simulink model "Testbed_v3"  (R2020a)
settings: Solver=ode23tb  StartTime=0.0  StopTime=20  MaxStep=0.066666666666666671  RelTol=1e-4  EnableMultiTasking=on
undefined symbols (not defined in the file): D11, Delta
libraries: powerlib x95, dspnetwork x75, dspstat3 x52, eePMU x16
(part 1 of 2)
settings Model: SimulationMode=accelerator  PacingRate=2000  Creator=vaibhav  LastModifiedBy=ray
settings SolverCC: MaxConsecutiveZCs=10000  ZeroCrossControl=EnableAll  ZeroCrossAlgorithm=Adaptive  SolverResetMethod=Robust
settings DataIOCC: LimitDataPoints=on  SaveFormat=Array  ReturnWorkspaceOutputs=off
settings OptimizationCC: ExpressionDepthLimit=2147483647  LifeSpan=inf
settings DebuggingCC: UnderspecifiedInitializationDetection=Classic  MergeDetectMultiDrivingBlocksExec=none  MaskedZcDiagnostic=none  IgnoredZcDiagnostic=none  SolverPrmCheckMsg=warning  FcnCallInpInsideContextMsg=warning  StateNameClashWarn=warning  SFUnexpectedBacktrackingDiag=warning  SFNoUnconditionalDefaultTransitionDiag=warning  SFExecutionAtInitializationDiag=none  ArithmeticOperatorsInVariantConditions=warning
settings HardwareCC: ProdBitPerPointer=32  ProdBitPerSizeT=32  ProdBitPerPtrDiffT=32  ProdLargestAtomicFloat=None  ProdIntDivRoundTo=Undefined  ProdEndianess=Unspecified  ProdWordSize=32  ProdHWDeviceType=32-bit Generic
settings ModelReferenceCC: PropagateSignalLabelsOutOfModel=off
settings SFSimCC: SimUseLocalCustomCode=off  CustomCodeUndefinedFunction=UseInterfaceOnly
settings RTWCC: RTWUseLocalCustomCode=off
settings CodeAppCC: StateflowObjectComments=on
settings GRTTargetCC: TargetLangStandard=C89/C90 (ANSI)  CombineOutputUpdateFcns=off  GRTInterface=on
settings ConfigComp: CovMetricSettings=dw  CovHtmlReporting=on  CovSaveCumulativeToWorkspaceVar=on  CovSaveSingleToWorkspaceVar=on  CovExternalEMLEnable=off

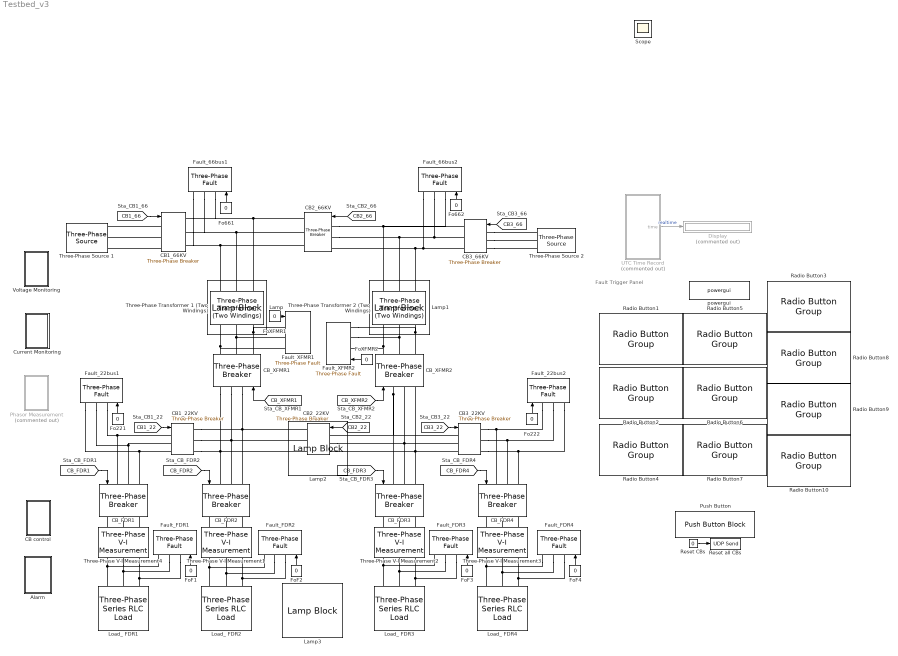
== system Testbed_v3 ==
  note: Fault Trigger
      | Panel
  Alarm : Subsystem
  CB control : Subsystem
  CB1_22KV : powerlib/Elements/Three-Phase Breaker  InitialState=closed  SwitchA=on  SwitchB=on  SwitchC=on  SwitchTimes="[1/10  2/10]"  External=on  BreakerResistance=0.0001  SnubberResistance=inf  SnubberCapacitance=inf  Measurements=Breaker voltages and currents
  CB1_66KV : powerlib/Elements/Three-Phase Breaker  InitialState=closed  SwitchA=on  SwitchB=on  SwitchC=on  SwitchTimes="[1/10  2/10]"  External=on  BreakerResistance=0.0001  SnubberResistance=inf  SnubberCapacitance=inf  Measurements=Breaker voltages and currents
  CB2_22KV : powerlib/Elements/Three-Phase Breaker  InitialState=closed  SwitchA=on  SwitchB=on  SwitchC=on  SwitchTimes="[1/10  2/10]"  External=on  BreakerResistance=0.0001  SnubberResistance=inf  SnubberCapacitance=inf  Measurements=Breaker voltages and currents
  CB2_66KV : powerlib/Elements/Three-Phase Breaker  InitialState=closed  SwitchA=on  SwitchB=on  SwitchC=on  SwitchTimes="[1/10  2/10]"  External=on  BreakerResistance=0.0001  SnubberResistance=inf  SnubberCapacitance=inf  Measurements=Breaker voltages and currents
  CB3_22KV : powerlib/Elements/Three-Phase Breaker  InitialState=closed  SwitchA=on  SwitchB=on  SwitchC=on  SwitchTimes="[1/10  2/10]"  External=on  BreakerResistance=0.0001  SnubberResistance=inf  SnubberCapacitance=inf  Measurements=Breaker voltages and currents
  CB3_66KV : powerlib/Elements/Three-Phase Breaker  InitialState=closed  SwitchA=on  SwitchB=on  SwitchC=on  SwitchTimes="[1/10  2/10]"  External=on  BreakerResistance=0.0001  SnubberResistance=inf  SnubberCapacitance=inf  Measurements=Breaker voltages and currents
  CB_FDR{1..4} (4 alike) : powerlib/Elements/Three-Phase Breaker  InitialState=closed  SwitchA=on  SwitchB=on  SwitchC=on  SwitchTimes="[1/10  2/10]"  External=on  BreakerResistance=0.0001  SnubberResistance=inf  SnubberCapacitance=inf  Measurements=Breaker voltages and currents
  CB_XFMR1 : powerlib/Elements/Three-Phase Breaker  InitialState=closed  SwitchA=on  SwitchB=on  SwitchC=on  SwitchTimes="[1/10  2/10]"  External=on  BreakerResistance=0.0001  SnubberResistance=inf  SnubberCapacitance=inf  Measurements=Breaker voltages and currents
  CB_XFMR2 : powerlib/Elements/Three-Phase Breaker  InitialState=closed  SwitchA=on  SwitchB=on  SwitchC=on  SwitchTimes="[1/10  2/10]"  External=on  BreakerResistance=0.0001  SnubberResistance=inf  SnubberCapacitance=inf  Measurements=Breaker voltages and currents
  Current Monitoring : Subsystem
  Display : Display  Commented=on
  Fault_22bus1 : powerlib/Elements/Three-Phase Fault  InitialStates=0  FaultA=on  FaultB=on  FaultC=on  GroundFault=off  SwitchTimes="[1/60  5/60]"  External=on  SwitchStatus=NaN  FaultResistance=0.0001  GroundResistance=0.01  SnubberResistance=inf  SnubberCapacitance=inf  Measurements=Fault voltages and currents
  Fault_22bus2 : powerlib/Elements/Three-Phase Fault  InitialStates=0  FaultA=on  FaultB=on  FaultC=on  GroundFault=off  SwitchTimes="[1/60  5/60]"  External=on  SwitchStatus=NaN  FaultResistance=0.0001  GroundResistance=0.01  SnubberResistance=inf  SnubberCapacitance=inf  Measurements=Fault voltages and currents
  Fault_66bus1 : powerlib/Elements/Three-Phase Fault  InitialStates=0  FaultA=on  FaultB=on  FaultC=on  GroundFault=off  SwitchTimes="[1/60  5/60]"  External=on  SwitchStatus=NaN  FaultResistance=0.0001  GroundResistance=0.01  SnubberResistance=inf  SnubberCapacitance=inf  Measurements=Fault voltages and currents
  Fault_66bus2 : powerlib/Elements/Three-Phase Fault  InitialStates=0  FaultA=on  FaultB=on  FaultC=on  GroundFault=off  SwitchTimes="[1/60  5/60]"  External=on  SwitchStatus=NaN  FaultResistance=0.0001  GroundResistance=0.01  SnubberResistance=inf  SnubberCapacitance=inf  Measurements=Fault voltages and currents
  Fault_FDR{1..4} (4 alike) : powerlib/Elements/Three-Phase Fault  InitialStates=0  FaultA=on  FaultB=on  FaultC=on  GroundFault=off  SwitchTimes="[1/60  5/60]"  External=on  SwitchStatus=NaN  FaultResistance=0.0001  GroundResistance=0.00001  SnubberResistance=inf  SnubberCapacitance=inf  Measurements=Fault voltages and currents
  Fault_XFMR1 : powerlib/Elements/Three-Phase Fault  InitialStates=0  FaultA=on  FaultB=on  FaultC=on  GroundFault=off  SwitchTimes="[1/60  5/60]"  External=on  SwitchStatus=NaN  FaultResistance=0.0001  GroundResistance=0.01  SnubberResistance=inf  SnubberCapacitance=inf  Measurements=Fault voltages and currents
  Fault_XFMR2 : powerlib/Elements/Three-Phase Fault  InitialStates=0  FaultA=on  FaultB=on  FaultC=on  GroundFault=off  SwitchTimes="[1/60  5/60]"  External=on  SwitchStatus=NaN  FaultResistance=0.0001  GroundResistance=0.01  SnubberResistance=inf  SnubberCapacitance=inf  Measurements=Fault voltages and currents
  Fo221 : Constant  Value=0  SampleTime=0
  Fo222 : Constant  Value=0  SampleTime=0
  Fo661 : Constant  Value=0  SampleTime=0
  Fo662 : Constant  Tag=fo662  Value=0  SampleTime=0
  FoF{1..4} (4 alike) : Constant  Value=0  SampleTime=0
  FoXFMR1 : Constant  Value=0  SampleTime=0
  FoXFMR2 : Constant  Value=0  SampleTime=0
  Lamp{,1..3} (4 alike) : LampBlock  LabelPosition=Hide
  Load_ FDR{1..4} (4 alike) : powerlib/Elements/Three-Phase Series RLC Load  LConnTagsString=A|B|C  Configuration=Delta  NominalVoltage=22000  Vabc=[1e3 1e3 1e3]  Vabcp=[1e3 1e3 1e3]  NominalFrequency=50  UnbalancedPower=off  ActivePower=1e6  InductivePower=100  CapacitivePower=100  Pabc=[10e3 9e3 11e3]  QLabc=[100 90 110]  QCabc=[100 90 110]  Pabcp=[10e3 9e3 11e3]  QLabcp=[100 90 110]  QCabcp=[100 90 110]  Measurements=Branch voltages and currents  LoadType=constant Z
  Phasor Measurement : Subsystem  Commented=on
  Push Button : PushButtonBlock  ButtonText=Reset All CBs
  Radio Button1 : RadioButtonGroup  LabelPosition=Hide  SelectedLabel=Normal  ButtonGroupName=Fault on 66bus1
      settings: Values={{'Normal', 'Short Circuit'}, [0 1]}
  Radio Button10 : RadioButtonGroup  LabelPosition=Hide  SelectedLabel=Normal  ButtonGroupName=Fault on FDR4
      settings: Values={{'Normal', 'Short Circuit'}, [0 1]}
  Radio Button2 : RadioButtonGroup  LabelPosition=Hide  SelectedLabel=Normal  ButtonGroupName=Fault on XFMR1
      settings: Values={{'Normal', 'Short Circuit'}, [0 1]}
  Radio Button3 : RadioButtonGroup  LabelPosition=Hide  SelectedLabel=Normal  ButtonGroupName=Fault on FDR1
      settings: Values={{'Normal', 'Short Circuit'}, [0 1]}
  Radio Button4 : RadioButtonGroup  LabelPosition=Hide  SelectedLabel=Normal  ButtonGroupName=Fault on 22BUS1
      settings: Values={{'Normal', 'Short Circuit'}, [0 1]}
  Radio Button5 : RadioButtonGroup  LabelPosition=Hide  SelectedLabel=Normal  ButtonGroupName=Fault on 66bus2
      settings: Values={{'Normal', 'Short Circuit'}, [0 1]}
  Radio Button6 : RadioButtonGroup  LabelPosition=Hide  SelectedLabel=Normal  ButtonGroupName=Fault on XFMR2
      settings: Values={{'Normal', 'Short Circuit'}, [0 1]}
  Radio Button7 : RadioButtonGroup  LabelPosition=Hide  SelectedLabel=Normal  ButtonGroupName=Fault on 22BUS2
      settings: Values={{'Normal', 'Short Circuit'}, [0 1]}
  Radio Button8 : RadioButtonGroup  LabelPosition=Hide  SelectedLabel=Normal  ButtonGroupName=Fault on FDR2
      settings: Values={{'Normal', 'Short Circuit'}, [0 1]}
  Radio Button9 : RadioButtonGroup  LabelPosition=Hide  SelectedLabel=Normal  ButtonGroupName=Fault on FDR3
      settings: Values={{'Normal', 'Short Circuit'}, [0 1]}
  Reset CBs : Constant  Value=0  SampleTime=0
  Reset all CBs : dspnetwork/UDP Send  remoteURL='23.23.23.255'  remotePort=10000  localURL='0.0.0.0'  localPortSource=Automatically determine  localPort=-1  sendBufferSize=8192  sampletime=-1  blockPlatform=[]  separateLengthPort=0
  Three-Phase Transformer 1 (Two Windings) : powerlib/Elements/Three-Phase Transformer (Two Windings)  Winding1Connection=Yg  Winding2Connection=Delta (D11)  CoreType=Three single-phase transformers  SetSaturation=off  Hysteresis=off  DataFile='hysteresis'  SetInitialFlux=off  Measurements=All measurements (V I Fluxes)  UNITS=pu  NominalPower=[ 25e6 , 50 ]  Winding1=[ 66e3 , 0.002 , 0.08 ]  Winding2=[ 22e3 , 0.002 , 0.08 ]  Rm=500  Lm=500  L0=0.5  Saturation=[ 0,0 ; 0.0024,1.2 ; 1.0,1.52 ]  InitialFluxes=[0.79999 -0.79999 0.69999]  BreakLoop=off  DiscreteSolver=Trapezoidal iterative  DataType=off  TransfoNumber=1
  Three-Phase Transformer 2 (Two Windings) : powerlib/Elements/Three-Phase Transformer (Two Windings)  Winding1Connection=Yg  Winding2Connection=Delta (D11)  CoreType=Three single-phase transformers  SetSaturation=off  Hysteresis=off  DataFile='hysteresis'  SetInitialFlux=off  Measurements=All measurements (V I Fluxes)  UNITS=pu  NominalPower=[ 25e6 , 50 ]  Winding1=[ 66e3 , 0.002 , 0.08 ]  Winding2=[ 22e3 , 0.002 , 0.08 ]  Rm=500  Lm=500  L0=0.5  Saturation=[ 0,0 ; 0.0024,1.2 ; 1.0,1.52 ]  InitialFluxes=[ 0.8 , -0.8 , 0.7 ]  BreakLoop=off  DiscreteSolver=Trapezoidal iterative  DataType=off  TransfoNumber=1
  Three-Phase V-I Measurement1 : powerlib/Measurements/Three-Phase V-I Measurement  VoltageMeasurement=phase-to-phase  SetLabelV=on  LabelV=Vfdr2  Vpu=off  VpuLL=off  CurrentMeasurement=yes  SetLabelI=on  LabelI=Ifdr2  Ipu=off  Pbase=100e6  Vbase=500e3  OutputType=Complex  PhasorSimulation=off  PSBequivalent=0
  Three-Phase V-I Measurement2 : powerlib/Measurements/Three-Phase V-I Measurement  VoltageMeasurement=phase-to-phase  SetLabelV=on  LabelV=Vfdr3  Vpu=off  VpuLL=off  CurrentMeasurement=yes  SetLabelI=on  LabelI=Ifdr3  Ipu=off  Pbase=100e6  Vbase=500e3  OutputType=Complex  PhasorSimulation=off  PSBequivalent=0
  Three-Phase V-I Measurement3 : powerlib/Measurements/Three-Phase V-I Measurement  VoltageMeasurement=phase-to-phase  SetLabelV=on  LabelV=Vfdr4  Vpu=off  VpuLL=off  CurrentMeasurement=yes  SetLabelI=on  LabelI=Ifdr4  Ipu=off  Pbase=100e6  Vbase=500e3  OutputType=Complex  PhasorSimulation=off  PSBequivalent=0
  Three-Phase V-I Measurement4 : powerlib/Measurements/Three-Phase V-I Measurement  VoltageMeasurement=phase-to-phase  SetLabelV=on  LabelV=Vfdr1  Vpu=off  VpuLL=off  CurrentMeasurement=yes  SetLabelI=on  LabelI=Ifdr1  Ipu=off  Pbase=100e6  Vbase=500e3  OutputType=Complex  PhasorSimulation=off  PSBequivalent=0
  Three-Phase Source 1 : powerlib/Electrical Sources/Three-Phase Source  InternalConnection=Yg  VoltagePhases=off  Voltage=66000  PhaseAngle=120  Voltage_phases=[66000 66000 66000]  PhaseAngles_phases=[0 -120 +120]  Frequency=50  NonIdealSource=off  SpecifyImpedance=off  Resistance=0.8929  Inductance=16.58e-3  ShortCircuitLevel=100e6  BaseVoltage=25e3  XRratio=7  BusType=swing  Pref=10e3  Qref=0  Prefabc=[10e3, 10e3, 10e3]  Qrefabc=[0, 0, 0]  Qmin=-inf  Qmax=inf
  Three-Phase Source 2 : powerlib/Electrical Sources/Three-Phase Source  InternalConnection=Yg  VoltagePhases=off  Voltage=66000  PhaseAngle=120  Voltage_phases=[114000 114000 114000]/sqrt(3)  PhaseAngles_phases=[0 -120 +120]  Frequency=50  NonIdealSource=off  SpecifyImpedance=off  Resistance=0.8929  Inductance=16.58e-3  ShortCircuitLevel=100e6  BaseVoltage=25e3  XRratio=7  BusType=swing  Pref=10e3  Qref=0  Prefabc=[10e3, 10e3, 10e3]  Qrefabc=[0, 0, 0]  Qmin=-inf  Qmax=inf
  UTC Time Record : MATLAB Function  Commented=on  TreatAsAtomicUnit=on
  Voltage Monitoring : Subsystem
  powergui : powerlib/powergui  Priority=1  SimulationMode=Continuous  SampleTime=50e-6  frequency=50  Iterations=50  frequencyindice=50  Pbase=100e6  ErrMax=1e-4  UnitsV=kV  UnitsW=MW  buscounter=0  FunctionMessages=off  echomessages=off  EnableUseOfTLC=off  CurrentSourceSwitches=off  DisableSnubberDevices=off  DisableRonSwitches=off  DisableVfSwitches=off  DisplayEquations=off  AutomaticDiscreteSolvers=off  SolverType=Tustin/Backward Euler (TBE)  Interpol=off  ExternalGateDelay=off  methode=off  Ts=100  x0status=blocks  SPID=off  SwTol=0  HookPort=off  NonlinearTolerance=1e-4  nMaxIteration=100  ContinueOnMaxIteration=off  RestoreLinks=warning  ResistiveCurrentMeasurement=off  Frange=[0:2:500]  Ylog=off  Xlog=on  ShowGrid=off  save=off  variable=ZData  structure=0  ZoomFFT=off  StartTime=0.0  cycles=1  DisplayStyle=1  fundamental=60  FreqAxis=off  MaxFrequency=1000  frequencyindicesteady=1  RmsSteady=1  display=off
  Scope : Scope
  wires:
  FoF4/1 -> Fault_FDR4/1
  FoXFMR1/1 -> Fault_XFMR1/1
  [CB_XFMR2] -> CB_XFMR2/1
  [CB3_66] -> CB3_66KV/1
  [CB2_66] -> CB2_66KV/1
  [CB2_22] -> CB2_22KV/1
  [CB1_66] -> CB1_66KV/1
  [CB_XFMR1] -> CB_XFMR1/1
  [CB_FDR1] -> CB_FDR1/1
  [CB_FDR2] -> CB_FDR2/1
  [CB_FDR3] -> CB_FDR3/1
  [CB_FDR4] -> CB_FDR4/1
  Fo662/1 -> Fault_66bus2/1
  Fo221/1 -> Fault_22bus1/1
  FoF3/1 -> Fault_FDR3/1
  FoF1/1 -> Fault_FDR1/1
  Fo661/1 -> Fault_66bus1/1
  FoXFMR2/1 -> Fault_XFMR2/1
  Fo222/1 -> Fault_22bus2/1
  [CB3_22] -> CB3_22KV/1
  [CB1_22] -> CB1_22KV/1
  FoF2/1 -> Fault_FDR2/1
  UTC Time Record/1(time) -> Display/1  "realtime"
  Reset CBs/1 -> Reset all CBs/1
  connections:
  CB_XFMR1/LConn3 -- CB1_22KV/RConn3 -- CB_FDR2/LConn1 -- CB2_22KV/RConn3
  CB_XFMR1/LConn2 -- CB1_22KV/RConn2 -- CB_FDR2/LConn2 -- CB2_22KV/RConn2
  CB_XFMR1/LConn1 -- CB1_22KV/RConn1 -- CB_FDR2/LConn3 -- CB2_22KV/RConn1
  CB_XFMR2/RConn1 -- Three-Phase Transformer 2 (Two Windings)/RConn1 -- Fault_XFMR2/LConn1
  CB_XFMR2/RConn3 -- Fault_XFMR2/LConn3 -- Three-Phase Transformer 2 (Two Windings)/RConn3
  CB_XFMR2/RConn2 -- Fault_XFMR2/LConn2 -- Three-Phase Transformer 2 (Two Windings)/RConn2
  CB3_66KV/LConn1 -- Three-Phase Source 2/RConn1
  CB3_66KV/LConn2 -- Three-Phase Source 2/RConn2
  CB3_66KV/LConn3 -- Three-Phase Source 2/RConn3
  CB2_66KV/LConn1 -- Fault_66bus2/LConn1 -- CB3_66KV/RConn1 -- Three-Phase Transformer 2 (Two Windings)/LConn1
  CB2_66KV/LConn2 -- Three-Phase Transformer 2 (Two Windings)/LConn2 -- Fault_66bus2/LConn2 -- CB3_66KV/RConn2
  CB3_66KV/RConn3 -- Fault_66bus2/LConn3 -- CB2_66KV/LConn3 -- Three-Phase Transformer 2 (Two Windings)/LConn3
  CB2_22KV/LConn2 -- CB3_22KV/LConn2 -- CB_FDR3/LConn2 -- CB_XFMR2/LConn2
  CB2_22KV/LConn3 -- CB3_22KV/LConn3 -- CB_FDR3/LConn3 -- CB_XFMR2/LConn3
  CB_XFMR2/LConn1 -- CB3_22KV/LConn1 -- CB_FDR3/LConn1 -- CB2_22KV/LConn1
  Three-Phase Transformer 1 (Two Windings)/LConn3 -- CB1_66KV/RConn3 -- Fault_66bus1/LConn3 -- CB2_66KV/RConn3
  Three-Phase Transformer 1 (Two Windings)/LConn2 -- Fault_66bus1/LConn2 -- CB1_66KV/RConn2 -- CB2_66KV/RConn2
  Three-Phase Transformer 1 (Two Windings)/LConn1 -- Fault_66bus1/LConn1 -- CB1_66KV/RConn1 -- CB2_66KV/RConn1
  CB_XFMR1/RConn3 -- Three-Phase Transformer 1 (Two Windings)/RConn3 -- Fault_XFMR1/LConn3
  CB_XFMR1/RConn2 -- Three-Phase Transformer 1 (Two Windings)/RConn2 -- Fault_XFMR1/LConn2
  CB_XFMR1/RConn1 -- Fault_XFMR1/LConn1 -- Three-Phase Transformer 1 (Two Windings)/RConn1
  CB1_66KV/LConn3 -- Three-Phase Source 1/RConn3
  CB1_66KV/LConn2 -- Three-Phase Source 1/RConn2
  CB1_66KV/LConn1 -- Three-Phase Source 1/RConn1
  Three-Phase V-I Measurement3/LConn2 -- CB_FDR4/RConn2
  Three-Phase V-I Measurement3/LConn3 -- CB_FDR4/RConn1
  Three-Phase V-I Measurement3/LConn1 -- CB_FDR4/RConn3
  Three-Phase V-I Measurement4/LConn2 -- CB_FDR1/RConn2
  Load_ FDR1/LConn2 -- Three-Phase V-I Measurement4/RConn2 -- Fault_FDR1/LConn2
  Three-Phase V-I Measurement4/LConn1 -- CB_FDR1/RConn3
  Three-Phase V-I Measurement4/LConn3 -- CB_FDR1/RConn1
  Load_ FDR1/LConn1 -- Three-Phase V-I Measurement4/RConn3 -- Fault_FDR1/LConn3
  Load_ FDR1/LConn3 -- Three-Phase V-I Measurement4/RConn1 -- Fault_FDR1/LConn1
  Three-Phase V-I Measurement1/LConn3 -- CB_FDR2/RConn1
  Three-Phase V-I Measurement1/LConn2 -- CB_FDR2/RConn2
  Three-Phase V-I Measurement1/LConn1 -- CB_FDR2/RConn3
  Load_ FDR3/LConn3 -- Fault_FDR3/LConn1 -- Three-Phase V-I Measurement2/RConn1
  Load_ FDR3/LConn2 -- Fault_FDR3/LConn2 -- Three-Phase V-I Measurement2/RConn2
  Load_ FDR3/LConn1 -- Fault_FDR3/LConn3 -- Three-Phase V-I Measurement2/RConn3
  Three-Phase V-I Measurement2/LConn3 -- CB_FDR3/RConn1
  Three-Phase V-I Measurement2/LConn2 -- CB_FDR3/RConn2
  Three-Phase V-I Measurement2/LConn1 -- CB_FDR3/RConn3
  Load_ FDR2/LConn1 -- Fault_FDR2/LConn3 -- Three-Phase V-I Measurement1/RConn3
  Load_ FDR2/LConn2 -- Fault_FDR2/LConn2 -- Three-Phase V-I Measurement1/RConn2
  Load_ FDR2/LConn3 -- Fault_FDR2/LConn1 -- Three-Phase V-I Measurement1/RConn1
  Load_ FDR4/LConn1 -- Fault_FDR4/LConn3 -- Three-Phase V-I Measurement3/RConn3
  Load_ FDR4/LConn2 -- Fault_FDR4/LConn2 -- Three-Phase V-I Measurement3/RConn2
  Load_ FDR4/LConn3 -- Fault_FDR4/LConn1 -- Three-Phase V-I Measurement3/RConn1
  CB3_22KV/RConn1 -- CB_FDR4/LConn1 -- Fault_22bus2/LConn1
  CB3_22KV/RConn2 -- CB_FDR4/LConn2 -- Fault_22bus2/LConn2
  CB3_22KV/RConn3 -- CB_FDR4/LConn3 -- Fault_22bus2/LConn3
  CB1_22KV/LConn1 -- Fault_22bus1/LConn1 -- CB_FDR1/LConn1
  CB1_22KV/LConn2 -- Fault_22bus1/LConn2 -- CB_FDR1/LConn2
  CB1_22KV/LConn3 -- Fault_22bus1/LConn3 -- CB_FDR1/LConn3

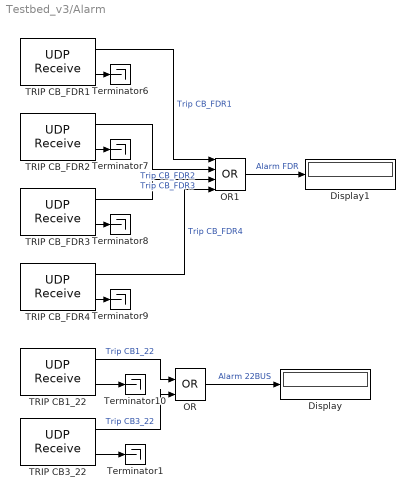
== system Testbed_v3/Alarm ==
  Display : Display
  Display1 : Display
  OR : Logic  Operator=OR  IconShape=distinctive  AllPortsSameDT=off  OutDataTypeStr=boolean
  OR1 : Logic  Operator=OR  Inputs=4  IconShape=distinctive  AllPortsSameDT=off  OutDataTypeStr=boolean
  TRIP CB1_22 : dspnetwork/UDP Receive  localURL='0.0.0.0'  localPort=22291  remoteURL='23.23.23.0'  remotePort=-1  recvBufferSize=2  dims=1  signalDatatype=uint16  isComplex=off  isVarSize=off  showBlockingTime=off  blockingTime=0  sampletime=0  blockPlatform=[]
  TRIP CB3_22 : dspnetwork/UDP Receive  localURL='0.0.0.0'  localPort=22293  remoteURL='23.23.23.0'  remotePort=-1  recvBufferSize=2  dims=1  signalDatatype=uint16  isComplex=off  isVarSize=off  showBlockingTime=off  blockingTime=0  sampletime=0  blockPlatform=[]
  TRIP CB_FDR1 : dspnetwork/UDP Receive  localURL='0.0.0.0'  localPort=21191  remoteURL='23.23.23.0'  remotePort=-1  recvBufferSize=2  dims=1  signalDatatype=uint16  isComplex=off  isVarSize=off  showBlockingTime=off  blockingTime=0  sampletime=0  blockPlatform=[]
  TRIP CB_FDR2 : dspnetwork/UDP Receive  localURL='0.0.0.0'  localPort=21192  remoteURL='23.23.23.0'  remotePort=-1  recvBufferSize=2  dims=1  signalDatatype=uint16  isComplex=off  isVarSize=off  showBlockingTime=off  blockingTime=0  sampletime=0  blockPlatform=[]
  TRIP CB_FDR3 : dspnetwork/UDP Receive  localURL='0.0.0.0'  localPort=21193  remoteURL='23.23.23.0'  remotePort=-1  recvBufferSize=2  dims=1  signalDatatype=uint16  isComplex=off  isVarSize=off  showBlockingTime=off  blockingTime=0  sampletime=0  blockPlatform=[]
  TRIP CB_FDR4 : dspnetwork/UDP Receive  localURL='0.0.0.0'  localPort=21194  remoteURL='23.23.23.0'  remotePort=-1  recvBufferSize=2  dims=1  signalDatatype=uint16  isComplex=off  isVarSize=off  showBlockingTime=off  blockingTime=0  sampletime=0  blockPlatform=[]
  Terminator{1,6..10} (6 alike) : Terminator
  wires:
  TRIP CB1_22/2 -> Terminator10/1
  TRIP CB3_22/2 -> Terminator1/1
  TRIP CB1_22/1 -> OR/1  "Trip CB1_22"
  TRIP CB3_22/1 -> OR/2  "Trip CB3_22"
  OR/1 -> Display/1  "Alarm 22BUS"
  TRIP CB_FDR4/2 -> Terminator9/1
  TRIP CB_FDR4/1 -> OR1/4  "Trip CB_FDR4"
  TRIP CB_FDR2/2 -> Terminator7/1
  TRIP CB_FDR1/1 -> OR1/1  "Trip CB_FDR1"
  TRIP CB_FDR2/1 -> OR1/2  "Trip CB_FDR2"
  TRIP CB_FDR3/1 -> OR1/3  "Trip CB_FDR3"
  TRIP CB_FDR3/2 -> Terminator8/1
  TRIP CB_FDR1/2 -> Terminator6/1
  OR1/1 -> Display1/1  "Alarm FDR"

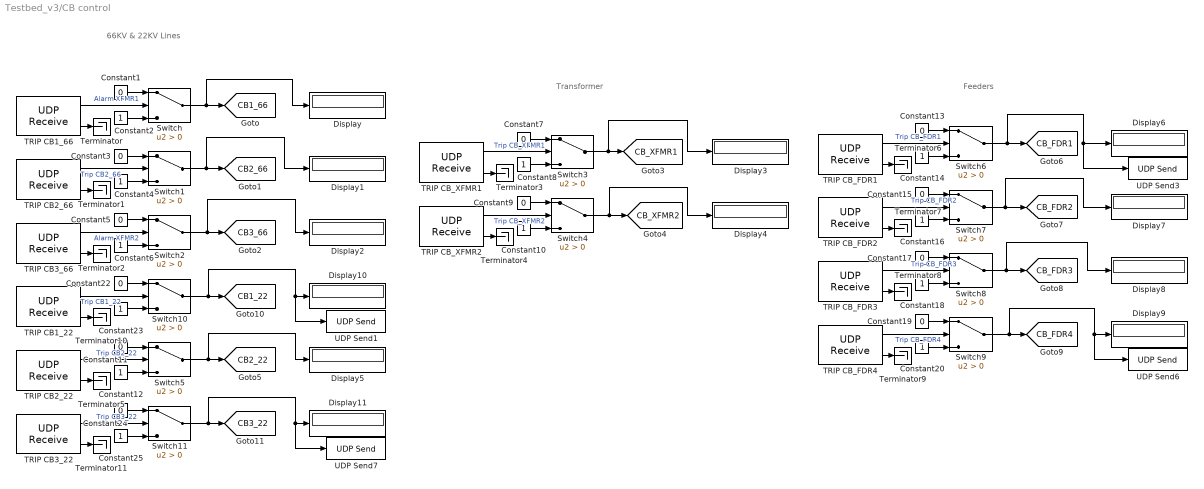
== system Testbed_v3/CB control ==
  note: 66KV & 22KV Lines
  note: Transformer
  note: Feeders
  Constant{1,3,5,7,9,11,13,15,17,19,22,24} (12 alike) : Constant  Value=0
  Constant{2,4,6,8,10,12,14,16,18,20,23,25} (12 alike) : Constant
  Display{,1..11} (12 alike) : Display
  Switch{,1..11} (12 alike) : Switch  Criteria=u2 > Threshold
  TRIP CB1_22 : dspnetwork/UDP Receive  localURL='0.0.0.0'  localPort=22291  remoteURL='23.23.23.0'  remotePort=-1  recvBufferSize=2  dims=1  signalDatatype=uint16  isComplex=off  isVarSize=off  showBlockingTime=off  blockingTime=0  sampletime=0  blockPlatform=[]
  TRIP CB1_66 : dspnetwork/UDP Receive  localURL='0.0.0.0'  localPort=26691  remoteURL='23.23.23.0'  remotePort=-1  recvBufferSize=2  dims=1  signalDatatype=uint16  isComplex=off  isVarSize=off  showBlockingTime=off  blockingTime=0  sampletime=0  blockPlatform=[]
  TRIP CB2_22 : dspnetwork/UDP Receive  localURL='0.0.0.0'  localPort=22292  remoteURL='23.23.23.0'  remotePort=-1  recvBufferSize=2  dims=1  signalDatatype=uint16  isComplex=off  isVarSize=off  showBlockingTime=off  blockingTime=0  sampletime=0  blockPlatform=[]
  TRIP CB2_66 : dspnetwork/UDP Receive  localURL='0.0.0.0'  localPort=26692  remoteURL='23.23.23.0'  remotePort=-1  recvBufferSize=2  dims=1  signalDatatype=uint16  isComplex=off  isVarSize=off  showBlockingTime=off  blockingTime=0  sampletime=0  blockPlatform=[]
  TRIP CB3_22 : dspnetwork/UDP Receive  localURL='0.0.0.0'  localPort=22293  remoteURL='23.23.23.0'  remotePort=-1  recvBufferSize=2  dims=1  signalDatatype=uint16  isComplex=off  isVarSize=off  showBlockingTime=off  blockingTime=0  sampletime=0  blockPlatform=[]
  TRIP CB3_66 : dspnetwork/UDP Receive  localURL='0.0.0.0'  localPort=26693  remoteURL='23.23.23.0'  remotePort=-1  recvBufferSize=2  dims=1  signalDatatype=uint16  isComplex=off  isVarSize=off  showBlockingTime=off  blockingTime=0  sampletime=0  blockPlatform=[]
  TRIP CB_FDR1 : dspnetwork/UDP Receive  localURL='0.0.0.0'  localPort=21191  remoteURL='23.23.23.0'  remotePort=-1  recvBufferSize=2  dims=1  signalDatatype=uint16  isComplex=off  isVarSize=off  showBlockingTime=off  blockingTime=0  sampletime=0  blockPlatform=[]
  TRIP CB_FDR2 : dspnetwork/UDP Receive  localURL='0.0.0.0'  localPort=21192  remoteURL='23.23.23.0'  remotePort=-1  recvBufferSize=2  dims=1  signalDatatype=uint16  isComplex=off  isVarSize=off  showBlockingTime=off  blockingTime=0  sampletime=0  blockPlatform=[]
  TRIP CB_FDR3 : dspnetwork/UDP Receive  localURL='0.0.0.0'  localPort=21193  remoteURL='23.23.23.0'  remotePort=-1  recvBufferSize=2  dims=1  signalDatatype=uint16  isComplex=off  isVarSize=off  showBlockingTime=off  blockingTime=0  sampletime=0  blockPlatform=[]
  TRIP CB_FDR4 : dspnetwork/UDP Receive  localURL='0.0.0.0'  localPort=21194  remoteURL='23.23.23.0'  remotePort=-1  recvBufferSize=2  dims=1  signalDatatype=uint16  isComplex=off  isVarSize=off  showBlockingTime=off  blockingTime=0  sampletime=0  blockPlatform=[]
  TRIP CB_XFMR1 : dspnetwork/UDP Receive  localURL='0.0.0.0'  localPort=23391  remoteURL='23.23.23.0'  remotePort=-1  recvBufferSize=2  dims=1  signalDatatype=uint16  isComplex=off  isVarSize=off  showBlockingTime=off  blockingTime=0  sampletime=0  blockPlatform=[]
  TRIP CB_XFMR2 : dspnetwork/UDP Receive  localURL='0.0.0.0'  localPort=23392  remoteURL='23.23.23.0'  remotePort=-1  recvBufferSize=2  dims=1  signalDatatype=uint16  isComplex=off  isVarSize=off  showBlockingTime=off  blockingTime=0  sampletime=0  blockPlatform=[]
  Terminator{,1..11} (12 alike) : Terminator
  UDP Send1 : dspnetwork/UDP Send  remoteURL='23.23.23.255'  remotePort=12291  localURL='0.0.0.0'  localPortSource=Automatically determine  localPort=-1  sendBufferSize=8192  sampletime=-1  blockPlatform=[]  separateLengthPort=0
  UDP Send3 : dspnetwork/UDP Send  remoteURL='23.23.23.255'  remotePort=11191  localURL='0.0.0.0'  localPortSource=Automatically determine  localPort=-1  sendBufferSize=8192  sampletime=-1  blockPlatform=[]  separateLengthPort=0
  UDP Send6 : dspnetwork/UDP Send  remoteURL='23.23.23.255'  remotePort=11194  localURL='0.0.0.0'  localPortSource=Automatically determine  localPort=-1  sendBufferSize=8192  sampletime=-1  blockPlatform=[]  separateLengthPort=0
  UDP Send7 : dspnetwork/UDP Send  remoteURL='23.23.23.255'  remotePort=12293  localURL='0.0.0.0'  localPortSource=Automatically determine  localPort=-1  sendBufferSize=8192  sampletime=-1  blockPlatform=[]  separateLengthPort=0
  tag scope: CB1_22=global, CB1_66=global, CB2_22=global, CB2_66=global, CB3_22=global, CB3_66=global, CB_FDR1=global, CB_FDR2=global, CB_FDR3=global, CB_FDR4=global, CB_XFMR1=global, CB_XFMR2=global
  wires:
  TRIP CB_XFMR1/1 -> Switch3/2  "Trip CB_XFMR1"
  TRIP CB2_66/1 -> Switch1/2  "Trip CB2_66"
  Constant8/1 -> Switch3/3
  Constant3/1 -> Switch1/1
  TRIP CB2_22/1 -> Switch5/2  "Trip CB2_22"
  TRIP CB_FDR1/2 -> Terminator6/1
  TRIP CB_FDR4/2 -> Terminator9/1
  Constant5/1 -> Switch2/1
  Constant17/1 -> Switch8/1
  TRIP CB_XFMR2/1 -> Switch4/2  "Trip CB_XFMR2"
  Constant12/1 -> Switch5/3
  TRIP CB_XFMR1/2 -> Terminator3/1
  Constant2/1 -> Switch/3
  Constant9/1 -> Switch4/1
  TRIP CB_FDR2/2 -> Terminator7/1
  Constant4/1 -> Switch1/3
  TRIP CB2_66/2 -> Terminator1/1
  TRIP CB1_66/1 -> Switch/2  "Alarm XFMR1"
  Constant6/1 -> Switch2/3
  TRIP CB_FDR3/2 -> Terminator8/1
  Constant13/1 -> Switch6/1
  Constant19/1 -> Switch9/1
  Constant20/1 -> Switch9/3
  TRIP CB_XFMR2/2 -> Terminator4/1
  TRIP CB1_66/2 -> Terminator/1
  Constant18/1 -> Switch8/3
  Switch/1 -> Display/1, [CB1_66]
  Constant7/1 -> Switch3/1
  TRIP CB2_22/2 -> Terminator5/1
  Constant11/1 -> Switch5/1
  Constant16/1 -> Switch7/3
  TRIP CB_FDR1/1 -> Switch6/2  "Trip CB_FDR1"
  TRIP CB_FDR3/1 -> Switch8/2  "Trip CB_FDR3"
  Constant10/1 -> Switch4/3
  TRIP CB_FDR2/1 -> Switch7/2  "Trip CB_FDR2"
  Constant14/1 -> Switch6/3
  Constant1/1 -> Switch/1
  Constant15/1 -> Switch7/1
  TRIP CB3_66/2 -> Terminator2/1
  TRIP CB_FDR4/1 -> Switch9/2  "Trip CB_FDR4"
  TRIP CB3_66/1 -> Switch2/2  "Alarm XFMR2"
  Switch1/1 -> Display1/1, [CB2_66]
  Switch2/1 -> Display2/1, [CB3_66]
  Switch5/1 -> Display5/1, [CB2_22]
  Switch3/1 -> Display3/1, [CB_XFMR1]
  Constant22/1 -> Switch10/1
  Constant23/1 -> Switch10/3
  TRIP CB1_22/2 -> Terminator10/1
  TRIP CB1_22/1 -> Switch10/2  "Trip CB1_22"
  Constant24/1 -> Switch11/1
  Constant25/1 -> Switch11/3
  TRIP CB3_22/2 -> Terminator11/1
  TRIP CB3_22/1 -> Switch11/2  "Trip CB3_22"
  Switch11/1 -> UDP Send7/1, Display11/1, [CB3_22]
  Switch4/1 -> Display4/1, [CB_XFMR2]
  Switch6/1 -> UDP Send3/1, Display6/1, [CB_FDR1]
  Switch7/1 -> Display7/1, [CB_FDR2]
  Switch8/1 -> Display8/1, [CB_FDR3]
  Switch9/1 -> UDP Send6/1, Display9/1, [CB_FDR4]
  Switch10/1 -> UDP Send1/1, Display10/1, [CB1_22]

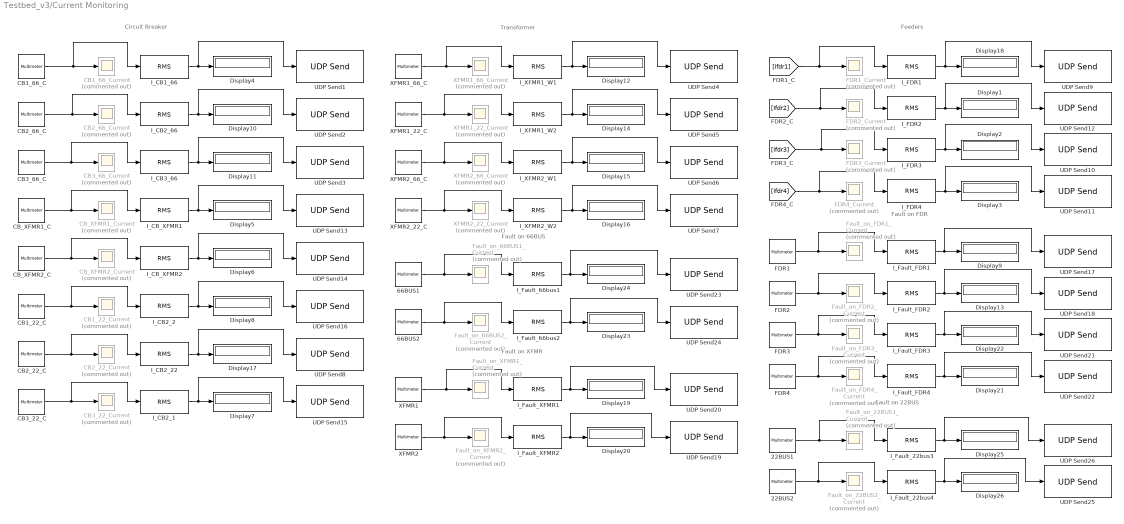
== system Testbed_v3/Current Monitoring ==
  note: Circuit Breaker
  note: Transformer
  note: Feeders
  note: Fault on XFMR
  note: Fault on FDR
  note: Fault on 66BUS
  note: Fault on 22BUS
  22BUS1 : powerlib/Measurements/Multimeter  PhasorSimulation=off  OutputType=Complex  sel=[139 140 141]  L=198  Gain=[1 1 1]  yselected={'Ib: Fault_22bus1/Fault A','Ib: Fault_22bus1/Fault B','Ib: Fault_22bus1/Fault C'};  PSBOutputType=1  PSBequivalent=0  AxesSetting=[0,0.1,-100,100]  Display=0  SavedBlockNames=-11
  22BUS2 : powerlib/Measurements/Multimeter  PhasorSimulation=off  OutputType=Complex  sel=[142 143 144]  L=198  Gain=[1 1 1]  yselected={'Ib: Fault_22bus2/Fault A','Ib: Fault_22bus2/Fault B','Ib: Fault_22bus2/Fault C'};  PSBOutputType=1  PSBequivalent=0  AxesSetting=[0,0.1,-100,100]  Display=0  SavedBlockNames=-11
  66BUS1 : powerlib/Measurements/Multimeter  PhasorSimulation=off  OutputType=Complex  sel=[145 146 147]  L=198  Gain=[1 1 1]  yselected={'Ib: Fault_66bus1/Fault A','Ib: Fault_66bus1/Fault B','Ib: Fault_66bus1/Fault C'};  PSBOutputType=1  PSBequivalent=0  AxesSetting=[0,0.1,-100,100]  Display=0  SavedBlockNames=-11
  66BUS2 : powerlib/Measurements/Multimeter  PhasorSimulation=off  OutputType=Complex  sel=[148 149 150]  L=198  Gain=[1 1 1]  yselected={'Ib: Fault_66bus2/Fault A','Ib: Fault_66bus2/Fault B','Ib: Fault_66bus2/Fault C'};  PSBOutputType=1  PSBequivalent=0  AxesSetting=[0,0.1,-100,100]  Display=0  SavedBlockNames=-11
  CB1_22_C : powerlib/Measurements/Multimeter  PhasorSimulation=off  OutputType=Complex  sel=[103 104 105]  L=198  Gain=[1 1 1]  yselected={'Ib: CB1_22KV/Breaker A','Ib: CB1_22KV/Breaker B','Ib: CB1_22KV/Breaker C'};  PSBOutputType=1  PSBequivalent=0  AxesSetting=[0,0.1,-100,100]  Display=0  SavedBlockNames=-11
  CB1_22_Current : Scope  Commented=on
  CB1_66_C : powerlib/Measurements/Multimeter  PhasorSimulation=off  OutputType=Complex  sel=[106 107 108]  L=198  Gain=[1 1 1]  yselected={'Ib: CB1_66KV/Breaker A','Ib: CB1_66KV/Breaker B','Ib: CB1_66KV/Breaker C'};  PSBOutputType=1  PSBequivalent=0  AxesSetting=[0,0.1,-100,100]  Display=0  SavedBlockNames=-11
  CB1_66_Current : Scope  Commented=on
  CB2_22_C : powerlib/Measurements/Multimeter  PhasorSimulation=off  OutputType=Complex  sel=[109 110 111]  L=198  Gain=[1 1 1]  yselected={'Ib: CB2_22KV/Breaker A','Ib: CB2_22KV/Breaker B','Ib: CB2_22KV/Breaker C'};  PSBOutputType=1  PSBequivalent=0  AxesSetting=[0,0.1,-100,100]  Display=0  SavedBlockNames=-11
  CB2_22_Current : Scope  Commented=on
  CB2_66_C : powerlib/Measurements/Multimeter  PhasorSimulation=off  OutputType=Complex  sel=[112 113 114]  L=198  Gain=[1 1 1]  yselected={'Ib: CB2_66KV/Breaker A','Ib: CB2_66KV/Breaker B','Ib: CB2_66KV/Breaker C'};  PSBOutputType=1  PSBequivalent=0  AxesSetting=[0,0.1,-100,100]  Display=0  SavedBlockNames=-11
  CB2_66_Current : Scope  Commented=on
  CB3_22_C : powerlib/Measurements/Multimeter  PhasorSimulation=off  OutputType=Complex  sel=[115 116 117]  L=198  Gain=[1 1 1]  yselected={'Ib: CB3_22KV/Breaker A','Ib: CB3_22KV/Breaker B','Ib: CB3_22KV/Breaker C'};  PSBOutputType=1  PSBequivalent=0  AxesSetting=[0,0.1,-100,100]  Display=0  SavedBlockNames=-11
  CB3_22_Current : Scope  Commented=on
  CB3_66_C : powerlib/Measurements/Multimeter  PhasorSimulation=off  OutputType=Complex  sel=[118 119 120]  L=198  Gain=[1 1 1]  yselected={'Ib: CB3_66KV/Breaker A','Ib: CB3_66KV/Breaker B','Ib: CB3_66KV/Breaker C'};  PSBOutputType=1  PSBequivalent=0  AxesSetting=[0,0.1,-100,100]  Display=0  SavedBlockNames=-11
  CB3_66_Current : Scope  Commented=on
  CB_XFMR1_C : powerlib/Measurements/Multimeter  PhasorSimulation=off  OutputType=Complex  sel=[133 134 135]  L=198  Gain=[1 1 1]  yselected={'Ib: CB_XFMR1/Breaker A','Ib: CB_XFMR1/Breaker B','Ib: CB_XFMR1/Breaker C'};  PSBOutputType=1  PSBequivalent=0  AxesSetting=[0,0.1,-100,100]  Display=0  SavedBlockNames=-11
  CB_XFMR1_Current : Scope  Commented=on
  CB_XFMR2_C : powerlib/Measurements/Multimeter  PhasorSimulation=off  OutputType=Complex  sel=[136 137 138]  L=198  Gain=[1 1 1]  yselected={'Ib: CB_XFMR2/Breaker A','Ib: CB_XFMR2/Breaker B','Ib: CB_XFMR2/Breaker C'};  PSBOutputType=1  PSBequivalent=0  AxesSetting=[0,0.1,-100,100]  Display=0  SavedBlockNames=-11
  CB_XFMR2_Current : Scope  Commented=on
  Display{1..26} (26 alike) : Display
  FDR1 : powerlib/Measurements/Multimeter  PhasorSimulation=off  OutputType=Complex  sel=[151 152 153]  L=198  Gain=[1 1 1]  yselected={'Ib: Fault_FDR1/Fault A','Ib: Fault_FDR1/Fault B','Ib: Fault_FDR1/Fault C'};  PSBOutputType=1  PSBequivalent=0  AxesSetting=[0,0.1,-100,100]  Display=0  SavedBlockNames=-11
  FDR1_Current : Scope  Commented=on
  FDR2 : powerlib/Measurements/Multimeter  PhasorSimulation=off  OutputType=Complex  sel=[154 155 156]  L=198  Gain=[1 1 1]  yselected={'Ib: Fault_FDR2/Fault A','Ib: Fault_FDR2/Fault B','Ib: Fault_FDR2/Fault C'};  PSBOutputType=1  PSBequivalent=0  AxesSetting=[0,0.1,-100,100]  Display=0  SavedBlockNames=-11
  FDR2_Current : Scope  Commented=on
  FDR3 : powerlib/Measurements/Multimeter  PhasorSimulation=off  OutputType=Complex  sel=[157 158 159]  L=198  Gain=[1 1 1]  yselected={'Ib: Fault_FDR3/Fault A','Ib: Fault_FDR3/Fault B','Ib: Fault_FDR3/Fault C'};  PSBOutputType=1  PSBequivalent=0  AxesSetting=[0,0.1,-100,100]  Display=0  SavedBlockNames=-11
  FDR3_Current : Scope  Commented=on
  FDR4 : powerlib/Measurements/Multimeter  PhasorSimulation=off  OutputType=Complex  sel=[160 161 162]  L=198  Gain=[1 1 1]  yselected={'Ib: Fault_FDR4/Fault A','Ib: Fault_FDR4/Fault B','Ib: Fault_FDR4/Fault C'};  PSBOutputType=1  PSBequivalent=0  AxesSetting=[0,0.1,-100,100]  Display=0  SavedBlockNames=-11
  FDR4_Current : Scope  Commented=on
  Fault_on_22BUS1_Current : Scope  Commented=on
  Fault_on_22BUS2_Current : Scope  Commented=on
  Fault_on_66BUS1_Current : Scope  Commented=on
  Fault_on_66BUS2_Current : Scope  Commented=on
  Fault_on_FDR1_Current : Scope  Commented=on
  Fault_on_FDR2_Current : Scope  Commented=on
  Fault_on_FDR3_Current : Scope  Commented=on
  Fault_on_FDR4_Current : Scope  Commented=on
  Fault_on_XFMR1_Current : Scope  Commented=on
  Fault_on_XFMR2_Current : Scope  Commented=on
  I_CB1_66 : dspstat3/RMS  run=off  directionMode=Specified dimension  dimension=1  reset_popup=None
  I_CB2_{1..2,22,66} (4 alike) : dspstat3/RMS  run=off  directionMode=Specified dimension  dimension=1  reset_popup=None
  I_CB3_66 : dspstat3/RMS  run=off  directionMode=Specified dimension  dimension=1  reset_popup=None
  I_CB_XFMR1 : dspstat3/RMS  run=off  directionMode=Specified dimension  dimension=1  reset_popup=None
  I_CB_XFMR2 : dspstat3/RMS  run=off  directionMode=Specified dimension  dimension=1  reset_popup=None
  I_FDR{1..4} (4 alike) : dspstat3/RMS  run=off  directionMode=Specified dimension  dimension=1  reset_popup=None
  I_Fault_22bus3 : dspstat3/RMS  run=off  directionMode=Specified dimension  dimension=1  reset_popup=None
  I_Fault_22bus4 : dspstat3/RMS  run=off  directionMode=Specified dimension  dimension=1  reset_popup=None
  I_Fault_66bus1 : dspstat3/RMS  run=off  directionMode=Specified dimension  dimension=1  reset_popup=None
  I_Fault_66bus2 : dspstat3/RMS  run=off  directionMode=Specified dimension  dimension=1  reset_popup=None
  I_Fault_FDR{1..4} (4 alike) : dspstat3/RMS  run=off  directionMode=Specified dimension  dimension=1  reset_popup=None
  I_Fault_XFMR1 : dspstat3/RMS  run=off  directionMode=Specified dimension  dimension=1  reset_popup=None
  I_Fault_XFMR2 : dspstat3/RMS  run=off  directionMode=Specified dimension  dimension=1  reset_popup=None
  I_XFMR1_W1 : dspstat3/RMS  run=off  directionMode=Specified dimension  dimension=1  reset_popup=None
  I_XFMR1_W2 : dspstat3/RMS  run=off  directionMode=Specified dimension  dimension=1  reset_popup=None
  I_XFMR2_W1 : dspstat3/RMS  run=off  directionMode=Specified dimension  dimension=1  reset_popup=None
  I_XFMR2_W2 : dspstat3/RMS  run=off  directionMode=Specified dimension  dimension=1  reset_popup=None
  UDP Send1 : dspnetwork/UDP Send  remoteURL='23.23.23.255'  remotePort=16611  localURL='0.0.0.0'  localPortSource=Automatically determine  localPort=-1  sendBufferSize=8192  sampletime=-1  blockPlatform=[]  separateLengthPort=0
  UDP Send10 : dspnetwork/UDP Send  remoteURL='23.23.23.255'  remotePort=11113  localURL='0.0.0.0'  localPortSource=Automatically determine  localPort=-1  sendBufferSize=8192  sampletime=-1  blockPlatform=[]  separateLengthPort=0
  UDP Send11 : dspnetwork/UDP Send  remoteURL='23.23.23.255'  remotePort=11114  localURL='0.0.0.0'  localPortSource=Automatically determine  localPort=-1  sendBufferSize=8192  sampletime=-1  blockPlatform=[]  separateLengthPort=0
  UDP Send12 : dspnetwork/UDP Send  remoteURL='23.23.23.255'  remotePort=11112  localURL='0.0.0.0'  localPortSource=Automatically determine  localPort=-1  sendBufferSize=8192  sampletime=-1  blockPlatform=[]  separateLengthPort=0
  UDP Send13 : dspnetwork/UDP Send  remoteURL='23.23.23.255'  remotePort=13311  localURL='0.0.0.0'  localPortSource=Automatically determine  localPort=-1  sendBufferSize=8192  sampletime=-1  blockPlatform=[]  separateLengthPort=0
  UDP Send14 : dspnetwork/UDP Send  remoteURL='23.23.23.255'  remotePort=13312  localURL='0.0.0.0'  localPortSource=Automatically determine  localPort=-1  sendBufferSize=8192  sampletime=-1  blockPlatform=[]  separateLengthPort=0
  UDP Send15 : dspnetwork/UDP Send  remoteURL='23.23.23.255'  remotePort=12213  localURL='0.0.0.0'  localPortSource=Automatically determine  localPort=-1  sendBufferSize=8192  sampletime=-1  blockPlatform=[]  separateLengthPort=0
  UDP Send16 : dspnetwork/UDP Send  remoteURL='23.23.23.255'  remotePort=12211  localURL='0.0.0.0'  localPortSource=Automatically determine  localPort=-1  sendBufferSize=8192  sampletime=-1  blockPlatform=[]  separateLengthPort=0
  UDP Send17 : dspnetwork/UDP Send  remoteURL='23.23.23.255'  remotePort=11141  localURL='0.0.0.0'  localPortSource=Automatically determine  localPort=-1  sendBufferSize=8192  sampletime=-1  blockPlatform=[]  separateLengthPort=0
  UDP Send18 : dspnetwork/UDP Send  remoteURL='23.23.23.255'  remotePort=11142  localURL='0.0.0.0'  localPortSource=Automatically determine  localPort=-1  sendBufferSize=8192  sampletime=-1  blockPlatform=[]  separateLengthPort=0
  UDP Send19 : dspnetwork/UDP Send  remoteURL='23.23.23.255'  remotePort=13342  localURL='0.0.0.0'  localPortSource=Automatically determine  localPort=-1  sendBufferSize=8192  sampletime=-1  blockPlatform=[]  separateLengthPort=0
  UDP Send2 : dspnetwork/UDP Send  remoteURL='23.23.23.255'  remotePort=16612  localURL='0.0.0.0'  localPortSource=Automatically determine  localPort=-1  sendBufferSize=8192  sampletime=-1  blockPlatform=[]  separateLengthPort=0
  UDP Send20 : dspnetwork/UDP Send  remoteURL='23.23.23.255'  remotePort=13341  localURL='0.0.0.0'  localPortSource=Automatically determine  localPort=-1  sendBufferSize=8192  sampletime=-1  blockPlatform=[]  separateLengthPort=0
  UDP Send21 : dspnetwork/UDP Send  remoteURL='23.23.23.255'  remotePort=11143  localURL='0.0.0.0'  localPortSource=Automatically determine  localPort=-1  sendBufferSize=8192  sampletime=-1  blockPlatform=[]  separateLengthPort=0
  UDP Send22 : dspnetwork/UDP Send  remoteURL='23.23.23.255'  remotePort=11144  localURL='0.0.0.0'  localPortSource=Automatically determine  localPort=-1  sendBufferSize=8192  sampletime=-1  blockPlatform=[]  separateLengthPort=0
  UDP Send23 : dspnetwork/UDP Send  remoteURL='23.23.23.255'  remotePort=16641  localURL='0.0.0.0'  localPortSource=Automatically determine  localPort=-1  sendBufferSize=8192  sampletime=-1  blockPlatform=[]  separateLengthPort=0
  UDP Send24 : dspnetwork/UDP Send  remoteURL='23.23.23.255'  remotePort=16642  localURL='0.0.0.0'  localPortSource=Automatically determine  localPort=-1  sendBufferSize=8192  sampletime=-1  blockPlatform=[]  separateLengthPort=0
  UDP Send25 : dspnetwork/UDP Send  remoteURL='23.23.23.255'  remotePort=12242  localURL='0.0.0.0'  localPortSource=Automatically determine  localPort=-1  sendBufferSize=8192  sampletime=-1  blockPlatform=[]  separateLengthPort=0
  UDP Send26 : dspnetwork/UDP Send  remoteURL='23.23.23.255'  remotePort=12241  localURL='0.0.0.0'  localPortSource=Automatically determine  localPort=-1  sendBufferSize=8192  sampletime=-1  blockPlatform=[]  separateLengthPort=0
  UDP Send3 : dspnetwork/UDP Send  remoteURL='23.23.23.255'  remotePort=16613  localURL='0.0.0.0'  localPortSource=Automatically determine  localPort=-1  sendBufferSize=8192  sampletime=-1  blockPlatform=[]  separateLengthPort=0
  UDP Send4 : dspnetwork/UDP Send  remoteURL='23.23.23.255'  remotePort=15511  localURL='0.0.0.0'  localPortSource=Automatically determine  localPort=-1  sendBufferSize=8192  sampletime=-1  blockPlatform=[]  separateLengthPort=0
  UDP Send5 : dspnetwork/UDP Send  remoteURL='23.23.23.255'  remotePort=14411  localURL='0.0.0.0'  localPortSource=Automatically determine  localPort=-1  sendBufferSize=8192  sampletime=-1  blockPlatform=[]  separateLengthPort=0
  UDP Send6 : dspnetwork/UDP Send  remoteURL='23.23.23.255'  remotePort=15512  localURL='0.0.0.0'  localPortSource=Automatically determine  localPort=-1  sendBufferSize=8192  sampletime=-1  blockPlatform=[]  separateLengthPort=0
  UDP Send7 : dspnetwork/UDP Send  remoteURL='23.23.23.255'  remotePort=14412  localURL='0.0.0.0'  localPortSource=Automatically determine  localPort=-1  sendBufferSize=8192  sampletime=-1  blockPlatform=[]  separateLengthPort=0
  UDP Send8 : dspnetwork/UDP Send  remoteURL='23.23.23.255'  remotePort=12212  localURL='0.0.0.0'  localPortSource=Automatically determine  localPort=-1  sendBufferSize=8192  sampletime=-1  blockPlatform=[]  separateLengthPort=0
  UDP Send9 : dspnetwork/UDP Send  remoteURL='23.23.23.255'  remotePort=11111  localURL='0.0.0.0'  localPortSource=Automatically determine  localPort=-1  sendBufferSize=8192  sampletime=-1  blockPlatform=[]  separateLengthPort=0
  XFMR1 : powerlib/Measurements/Multimeter  PhasorSimulation=off  OutputType=Complex  sel=[163 164 165]  L=198  Gain=[1 1 1]  yselected={'Ib: Fault_XFMR1/Fault A','Ib: Fault_XFMR1/Fault B','Ib: Fault_XFMR1/Fault C'};  PSBOutputType=1  PSBequivalent=0  AxesSetting=[0,0.1,-100,100]  Display=0  SavedBlockNames=-11
  XFMR1_22_C : powerlib/Measurements/Multimeter  PhasorSimulation=off  OutputType=Complex  sel=[172 173 174]  L=198  Gain=[1 1 1]  yselected={'Iab_w2: Three-Phase Transformer 1 (Two Windings)','Ibc_w2: Three-Phase Transformer 1 (Two Windings)','Ica_w2: Three-Phase Transformer 1 (Two Windings)'};  PSBOutputType=1  PSBequivalent=0  AxesSetting=[0,0.1,-100,100]  Display=0  SavedBlockNames=-11
  XFMR1_22_Current : Scope  Commented=on
  XFMR1_66_C : powerlib/Measurements/Multimeter  PhasorSimulation=off  OutputType=Complex  sel=[169 170 171]  L=198  Gain=[1 1 1]  yselected={'Iag_w1: Three-Phase Transformer 1 (Two Windings)','Ibg_w1: Three-Phase Transformer 1 (Two Windings)','Icg_w1: Three-Phase Transformer 1 (Two Windings)'};  PSBOutputType=1  PSBequivalent=0  AxesSetting=[0,0.1,-100,100]  Display=0  SavedBlockNames=-11
  XFMR1_66_Current : Scope  Commented=on
  XFMR2 : powerlib/Measurements/Multimeter  PhasorSimulation=off  OutputType=Complex  sel=[166 167 168]  L=198  Gain=[1 1 1]  yselected={'Ib: Fault_XFMR2/Fault A','Ib: Fault_XFMR2/Fault B','Ib: Fault_XFMR2/Fault C'};  PSBOutputType=1  PSBequivalent=0  AxesSetting=[0,0.1,-100,100]  Display=0  SavedBlockNames=-11
  XFMR2_22_C : powerlib/Measurements/Multimeter  PhasorSimulation=off  OutputType=Complex  sel=[178 179 180]  L=198  Gain=[1 1 1]  yselected={'Iab_w2: Three-Phase Transformer 2 (Two Windings)','Ibc_w2: Three-Phase Transformer 2 (Two Windings)','Ica_w2: Three-Phase Transformer 2 (Two Windings)'};  PSBOutputType=1  PSBequivalent=0  AxesSetting=[0,0.1,-100,100]  Display=0  SavedBlockNames=-11
  XFMR2_22_Current : Scope  Commented=on
  XFMR2_66_C : powerlib/Measurements/Multimeter  PhasorSimulation=off  OutputType=Complex  sel=[175 176 177]  L=198  Gain=[1 1 1]  yselected={'Iag_w1: Three-Phase Transformer 2 (Two Windings)','Ibg_w1: Three-Phase Transformer 2 (Two Windings)','Icg_w1: Three-Phase Transformer 2 (Two Windings)'};  PSBOutputType=1  PSBequivalent=0  AxesSetting=[0,0.1,-100,100]  Display=0  SavedBlockNames=-11
  XFMR2_66_Current : Scope  Commented=on
  wires:
  I_CB1_66/1 -> UDP Send1/1, Display4/1
  I_CB2_66/1 -> UDP Send2/1, Display10/1
  I_FDR3/1 -> UDP Send10/1, Display2/1
  CB3_66_C/1 -> I_CB3_66/1, CB3_66_Current/1
  I_XFMR2_W1/1 -> UDP Send6/1, Display15/1
  I_FDR1/1 -> UDP Send9/1, Display18/1
  I_XFMR1_W1/1 -> UDP Send4/1, Display12/1
  I_FDR2/1 -> UDP Send12/1, Display1/1
  I_XFMR2_W2/1 -> UDP Send7/1, Display16/1
  I_FDR4/1 -> UDP Send11/1, Display3/1
  I_CB3_66/1 -> UDP Send3/1, Display11/1
  [Ifdr1] -> I_FDR1/1, FDR1_Current/1
  XFMR2_22_C/1 -> I_XFMR2_W2/1, XFMR2_22_Current/1
  [Ifdr2] -> I_FDR2/1, FDR2_Current/1
  CB2_66_C/1 -> I_CB2_66/1, CB2_66_Current/1
  [Ifdr4] -> I_FDR4/1, FDR4_Current/1
  XFMR1_22_C/1 -> I_XFMR1_W2/1, XFMR1_22_Current/1
  CB1_66_C/1 -> I_CB1_66/1, CB1_66_Current/1
  XFMR2_66_C/1 -> I_XFMR2_W1/1, XFMR2_66_Current/1
  [Ifdr3] -> I_FDR3/1, FDR3_Current/1
  I_XFMR1_W2/1 -> UDP Send5/1, Display14/1
  I_CB_XFMR1/1 -> UDP Send13/1, Display5/1
  CB_XFMR1_C/1 -> I_CB_XFMR1/1, CB_XFMR1_Current/1
  I_CB_XFMR2/1 -> UDP Send14/1, Display6/1
  CB_XFMR2_C/1 -> I_CB_XFMR2/1, CB_XFMR2_Current/1
  XFMR1_66_C/1 -> I_XFMR1_W1/1, XFMR1_66_Current/1
  FDR2/1 -> I_Fault_FDR2/1, Fault_on_FDR2_Current/1
  FDR1/1 -> I_Fault_FDR1/1, Fault_on_FDR1_Current/1
  I_Fault_FDR1/1 -> UDP Send17/1, Display9/1
  I_Fault_FDR2/1 -> UDP Send18/1, Display13/1
  I_Fault_XFMR2/1 -> UDP Send19/1, Display20/1
  XFMR1/1 -> I_Fault_XFMR1/1, Fault_on_XFMR1_Current/1
  XFMR2/1 -> I_Fault_XFMR2/1, Fault_on_XFMR2_Current/1
  I_Fault_XFMR1/1 -> UDP Send20/1, Display19/1
  I_Fault_FDR3/1 -> UDP Send21/1, Display22/1
  FDR3/1 -> I_Fault_FDR3/1, Fault_on_FDR3_Current/1
  FDR4/1 -> I_Fault_FDR4/1, Fault_on_FDR4_Current/1
  I_Fault_FDR4/1 -> UDP Send22/1, Display21/1
  I_Fault_66bus1/1 -> UDP Send23/1, Display24/1
  66BUS1/1 -> I_Fault_66bus1/1, Fault_on_66BUS1_Current/1
  66BUS2/1 -> I_Fault_66bus2/1, Fault_on_66BUS2_Current/1
  I_Fault_66bus2/1 -> UDP Send24/1, Display23/1
  I_Fault_22bus3/1 -> UDP Send26/1, Display25/1
  I_Fault_22bus4/1 -> UDP Send25/1, Display26/1
  22BUS2/1 -> I_Fault_22bus4/1, Fault_on_22BUS2_Current/1
  22BUS1/1 -> I_Fault_22bus3/1, Fault_on_22BUS1_Current/1
  I_CB2_22/1 -> UDP Send8/1, Display17/1
  CB2_22_C/1 -> I_CB2_22/1, CB2_22_Current/1
  CB3_22_C/1 -> I_CB2_1/1, CB3_22_Current/1
  I_CB2_1/1 -> UDP Send15/1, Display7/1
  CB1_22_C/1 -> I_CB2_2/1, CB1_22_Current/1
  I_CB2_2/1 -> UDP Send16/1, Display8/1
